simulink model "advisordemo1"  (Simulink 5.0)
settings: Solver=VariableStepDiscrete  SolverMode=SingleTasking  StartTime=0.0  StopTime=4  FixedStep=1  RelTol=1e-3  AbsTol=1e-6
libraries: fixpt_lib_4 x1, simulink x1
settings Model: ExecutionOrder=on  CovMetricSettings=d  Creator=andyb  LastModifiedBy=batserve  ExtModeTrigMode=oneshot  ExtModeArmWhenConnect=off  ExtModeAutoUpdateStatusClock=off  SaveState=on  SaveOutput=off  SaveFinalState=on  LimitDataPoints=off  IntegerOverflowMsg=none  ParameterDowncastMsg=warning  ParameterOverflowMsg=warning  ParameterPrecisionLossMsg=none  BlockReductionOpt=off  BooleanDataType=off  ConditionallyExecuteInputs=off  ParameterPooling=off  OptimizeBlockIOStorage=off  ProdHWWordLengths=8,16,16,32  RTWSystemTargetFile=ert.tlc  RTWTemplateMakefile=ert_default_tmf  RTWGenerateCodeOnly=on  RTWOptions="-aCombineOutputUpdateFcns=1 -aEnforceIntegerDowncast=0 -aExtMode=1 -aExtModeTesting=0 -aFoldNonRolledExpr=0 -aForceParamTrailComments=0 -aGenFloatMathFcnCalls=\"ANSI_C\" -aGenerateASAP2=0 -aGenerateComments=0 -aGenerateErtSFunction=0 -aGenerateReport=0 -aGenerateSampleERTMain=1 -aIgnoreCustomStorageClasses=0 -aIncDataTypeInIds=1 -aIncHierarchyInIds=1 -aIncludeMdlTerminateFcn=1 -aInitFltsAndDblsToZero=1 -aInlineInvariantSignals=0 -aInlinedPrmAccess=\"Literals\" -aInsertBlockDesc=0 -aLocalBlockOutputs=0 -aMatFileLogging=0 -aMaxRTWIdLen=31 -aMultiInstanceERTCode=0 -aPrefixModelToSubsysFcnNames=1 -aPurelyIntegerCode=0 -aRTWVerbose=1 -aRollThreshold=5 -aShowEliminatedStatements=0 -aSuppressErrorStatus=0 -aTargetOS=\"BareBoardExample\" -aZeroExternalMemoryAtStartup=1 -aZeroInternalMemoryAtStartup=1"

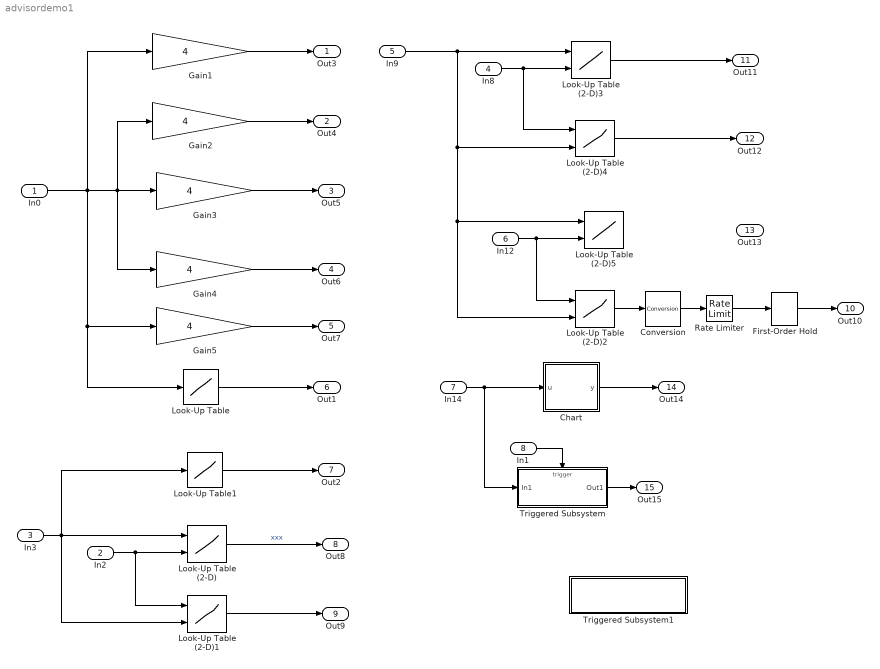
== system advisordemo1 ==
  In0 : Inport  ShowAdditionalParam=on  DataType=Specify via dialog  OutDataType=sfix(8)  OutScaling=2^-4  Interpolate=off
  In2 : Inport  Port=2  ShowAdditionalParam=on  DataType=Specify via dialog  OutScaling=2^-10  Interpolate=off
  In3 : Inport  Port=3  ShowAdditionalParam=on  DataType=Specify via dialog  OutScaling=2^-10  Interpolate=off
  In8 : Inport  Port=4  ShowAdditionalParam=on  DataType=Specify via dialog  OutScaling=2^-10  Interpolate=off
  In9 : Inport  Port=5  ShowAdditionalParam=on  DataType=Specify via dialog  OutScaling=2^-10  Interpolate=off
  In12 : Inport  Port=6  ShowAdditionalParam=on  DataType=Specify via dialog  OutScaling=2^-10  Interpolate=off
  In14 : Inport  Port=7  ShowAdditionalParam=on  OutScaling=2^-10  Interpolate=off
  In1 : Inport  Port=8  ShowAdditionalParam=on  DataType=boolean  OutScaling=2^-10  Interpolate=off
  Chart : Stateflow chart
  Conversion : fixpt_lib_4/Data Type/Conversion  ConvertRealWorld=Stored Integer  OutDataType=sfix(16)  OutScaling=2^-10  DoSatur=off
  First-Order Hold : simulink/Discrete/First-Order Hold  Ts=1
  Gain1 : Gain  Gain=4  ShowAdditionalParam=on  ParameterScaling=2^-15  OutScaling=2^-10
  Gain2 : Gain  Gain=4  ShowAdditionalParam=on  ParameterDataTypeMode=Specify via dialog  ParameterDataType=sfix(32)  ParameterScalingMode=Use specified scaling  OutScaling=2^-10  SaturateOnIntegerOverflow=on
  Gain3 : Gain  Gain=4  ShowAdditionalParam=on  ParameterDataTypeMode=Specify via dialog  ParameterDataType=sfix(32)  ParameterScalingMode=Use specified scaling  OutScaling=2^-10
  Gain4 : Gain  Gain=4  ShowAdditionalParam=on  ParameterDataTypeMode=Specify via dialog  ParameterDataType=sfix(32)  ParameterScalingMode=Use specified scaling  OutDataTypeMode=Specify via dialog  OutDataType=sfix(32)  OutScaling=2^-4
  Gain5 : Gain  Gain=4  ShowAdditionalParam=on  ParameterDataTypeMode=Specify via dialog  ParameterDataType=sfix(32)  ParameterScalingMode=Use specified scaling  OutDataTypeMode=Specify via dialog  OutDataType=sfix(32)  OutScaling=2^-3  SaturateOnIntegerOverflow=on
  Look-Up Table : Lookup  InputValues=[0 1 3 7]  OutputValues=[9 3 9 3]  ShowAdditionalParam=on  LookUpMeth=Interpolation-Use End Values  OutDataTypeMode=Specify via dialog  OutScaling=2^-10  RndMeth=Nearest
  Look-Up Table (2-D) : Lookup2D  RowIndex=[1:3]  ColumnIndex=[1:3]  OutputValues=[4 5 6;16 19 20;10 18 23]  ShowAdditionalParam=on  LookUpMeth=Interpolation-Use End Values  OutDataTypeMode=Specify via dialog  OutScaling=2^-10
  Look-Up Table (2-D)1 : Lookup2D  RowIndex=[0 2 5]  ColumnIndex=[1:3]  OutputValues=[4 5 6;16 19 20;10 18 23]  ShowAdditionalParam=on  LookUpMeth=Interpolation-Use End Values  OutDataTypeMode=Specify via dialog  OutScaling=2^-10
  Look-Up Table (2-D)2 : Lookup2D  RowIndex=[1:3]  ColumnIndex=[1 2 7]  OutputValues=[4 5 6;16 19 20;10 18 23]  ShowAdditionalParam=on  LookUpMeth=Interpolation-Use End Values  OutDataTypeMode=Specify via dialog  OutScaling=2^-10
  Look-Up Table (2-D)3 : Lookup2D  RowIndex=[1:3]  ColumnIndex=[20 20.05 20.1]  OutputValues=[4 5 6;16 19 20;10 18 23]  ShowAdditionalParam=on  LookUpMeth=Interpolation-Use End Values  OutDataTypeMode=Specify via dialog  OutScaling=2^-10
  Look-Up Table (2-D)4 : Lookup2D  RowIndex=[1:3]  ColumnIndex=[20.00 20.05 20.10 20.15 20.20]  OutputValues=ones(3,5)  ShowAdditionalParam=on  LookUpMeth=Interpolation-Use End Values  OutDataTypeMode=Specify via dialog  OutScaling=2^-10
  Look-Up Table (2-D)5 : Lookup2D  RowIndex=[20.00 20.05 20.10 20.15 20.20]  ColumnIndex=[1:3]  OutputValues=ones(3,5).'  ShowAdditionalParam=on  LookUpMeth=Interpolation-Use End Values  OutDataTypeMode=Specify via dialog  OutScaling=2^-10
  Look-Up Table1 : Lookup  InputValues=[20 20.05 20.1 20.15 20.2]  OutputValues=[9 3 9 3 9]  ShowAdditionalParam=on  LookUpMeth=Interpolation-Use End Values  OutDataTypeMode=Specify via dialog  OutScaling=2^-10
  Rate Limiter : RateLimiter
  Triggered Subsystem : Subsystem  TreatAsAtomicUnit=on
  Triggered Subsystem1 : Subsystem
      mask Display: disp('Read Me . . .')
  Out3 : Outport
  Out4 : Outport  Port=2
  Out5 : Outport  Port=3
  Out6 : Outport  Port=4
  Out7 : Outport  Port=5
  Out1 : Outport  Port=6
  Out2 : Outport  Port=7
  Out8 : Outport  Port=8
  Out9 : Outport  Port=9
  Out10 : Outport  Port=10
  Out11 : Outport  Port=11
  Out12 : Outport  Port=12
  Out13 : Outport  Port=13
  Out14 : Outport  Port=14
  Out15 : Outport  Port=15
  wires:
  Gain1/1 -> Out3/1
  Gain2/1 -> Out4/1
  Gain3/1 -> Out5/1
  Gain4/1 -> Out6/1
  Gain5/1 -> Out7/1
  Look-Up Table/1 -> Out1/1
  Look-Up Table1/1 -> Out2/1
  In2/1 -> Look-Up Table (2-D)/2, Look-Up Table (2-D)1/1
  Look-Up Table (2-D)/1 -> Out8/1  "xxx"
  In3/1 -> Look-Up Table (2-D)/1, Look-Up Table (2-D)1/2, Look-Up Table1/1
  Look-Up Table (2-D)1/1 -> Out9/1
  Look-Up Table (2-D)2/1 -> Conversion/1
  In8/1 -> Look-Up Table (2-D)3/2, Look-Up Table (2-D)4/1
  Look-Up Table (2-D)3/1 -> Out11/1
  In9/1 -> Look-Up Table (2-D)3/1, Look-Up Table (2-D)4/2, Look-Up Table (2-D)5/1, Look-Up Table (2-D)2/2
  Look-Up Table (2-D)4/1 -> Out12/1
  In12/1 -> Look-Up Table (2-D)5/2, Look-Up Table (2-D)2/1
  Rate Limiter/1 -> First-Order Hold/1
  Conversion/1 -> Rate Limiter/1
  First-Order Hold/1 -> Out10/1
  In14/1 -> Chart/1(u), Triggered Subsystem/1(In1)
  Chart/1(y) -> Out14/1
  In0/1 -> Gain3/1, Gain4/1, Gain2/1, Gain1/1, Gain5/1, Look-Up Table/1
  Triggered Subsystem/1(Out1) -> Out15/1
  In1/1 -> Triggered Subsystem/Trigger

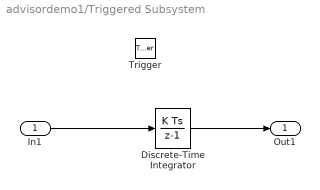
== system advisordemo1/Triggered Subsystem ==
  In1 : Inport
  Trigger : TriggerPort
  Discrete-Time Integrator : DiscreteIntegrator  SampleTime=-1
  Out1 : Outport
  wires:
  In1/1 -> Discrete-Time Integrator/1
  Discrete-Time Integrator/1 -> Out1/1

== system advisordemo1/Triggered Subsystem1 ==
  note: Recommended usage of the Model Assistant Tool
  note: 1.  Select the appropriate system target file prior to using the Model Assistant Tool.
      | This demo model is pre-configured for grt.tlc to illustrate functionality of the Model
      | Advisor component.  Generally speaking, you should first select ert.tlc, or an
      | appropriate ERT-based target (such as mpc555_exp.tlc).
      |
      | 2. Invoke the Model Assistant Tool from MATLAB: modelassistant('advisordemo1')
      |
      | 3. Run the High-Level Configuration component.
      |
      | 4. Run the Model Advisor component, and address any reported issues.
      |
      | 5. Adjust specific options using the Detailed Configuration component
      |
      | Note that the Search and Modify component is a useful tool for performing
      | batch operations.

== stateflow chart Chart ==
  state B
  state A
  A -> B : {y=u*2;}
  (default) -> A
  data: u input int32; y output int32
